simulink model "MOTOR2"  (Simulink 5.1)
settings: Solver=ode45  StartTime=0.0  StopTime=10.0  RelTol=1e-3
settings Model: LastModifiedBy=esposito  ExtModeTrigMode=oneshot  ExtModeArmWhenConnect=off  LimitDataPoints=off  ProdHWDeviceType=Microprocessor

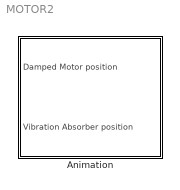
== system MOTOR2 ==
  Animation : Subsystem

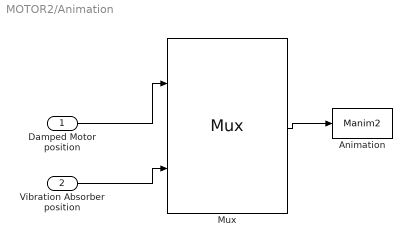
== system MOTOR2/Animation ==
  Damped Motor position : Inport
  Vibration Absorber position : Inport  Port=2
  Animation : S-Function  FunctionName=Manim2
  Mux : Mux  Inputs=2
  wires:
  Damped Motor position/1 -> Mux/1
  Vibration Absorber position/1 -> Mux/2
  Mux/1 -> Animation/1
